simulink model "untitled"  (R2018a)
settings: Solver=VariableStepAuto  StartTime=0.0  StopTime=inf  RelTol=1e-3
libraries: simulink_extras x1, simulink x1
settings Model: Creator=sajan.gict16  LastModifiedBy=sajan.gict16

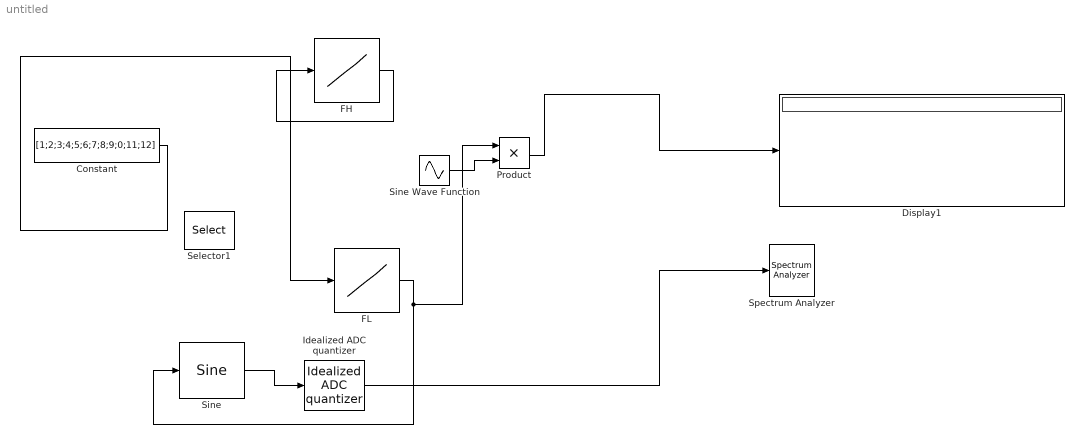
== system untitled ==
  Constant : Constant  Value=[1;2;3;4;5;6;7;8;9;0;11;12]
  Display1 : Display
  FH : Lookup_n-D  NumberOfTableDimensions=1  BreakpointsForDimension1=[0,1,2,3,4,5,6,7,8,9,11,12]  Table=[1209,1209,1209,1209,1336,1336,1336,1336,1477,1477,1477,1477]  InternalRulePriority=Speed  RndMeth=Simplest  InputSameDT=on
  "FL " : Lookup_n-D  NumberOfTableDimensions=1  BreakpointsForDimension1=[0,1,2,3,4,5,6,7,8,9,11,12]  Table=[697,770,852,941,697,770,852,941,697,770,852,941]  InternalRulePriority=Speed  RndMeth=Simplest  InputSameDT=on
  Idealized ADC quantizer : simulink_extras/Additional Discrete/Idealized ADC quantizer  NumberOfConverterBits=32  Vmin=0  Vmax=5  OutputDataType=int16  OutputNegativeValues=off
      settings: SourceProductName=Simulink
  Product : Product
  Selector1 : Selector  NumberOfDimensions=12  IndexMode=Zero-based  InputPortWidth=3  IndexOptions=Index vector (dialog),Index vector (dialog),Index vector (dialog),Index vector (dialog),Index vector (dialog),Index vector (dialog),Index vector (dialog),Index vector (dialog),Index vector (dialog),Index vector (dialog),Index vector (dialog),Index vector (dialog)  Indices=0,1,2,3,4,5,6,7,8,9,11,12  OutputSizes=1,1,1,1,1,1,1,1,1,1,1,1
  Sine : simulink/Lookup Tables/Sine  Formula=sin(2*pi*u)  NumDataPoints=12  OutputWordLength=16  InternalRulePriority=Speed
      settings: SourceProductName=Simulink
  Sine Wave Function : Sin  SineType=Sample based  Samples=100  SampleTime=1
  Spectrum Analyzer : SpectrumAnalyzer
  wires:
  Product/1 -> Display1/1
  Constant/1 -> "FL "/1
  Sine Wave Function/1 -> Product/2
  FH/1 -> FH/1
  "FL "/1 -> Product/1, Sine/1
  Sine/1 -> Idealized ADC quantizer/1
  Idealized ADC quantizer/1 -> Spectrum Analyzer/1
